simulink model "InAmpCode"  (R2025b)
settings: Solver=VariableStepAuto  StartTime=0.0  StopTime=10  RelTol=1e-3
libraries: fl_lib x15, nesl_utility x3
settings Model: Creator=Bassel  LastModifiedBy=Bassel

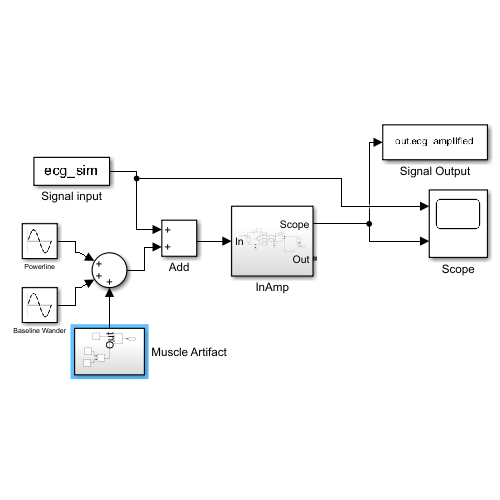
[thumbnail: Simulink's stored preview of the top-level diagram]
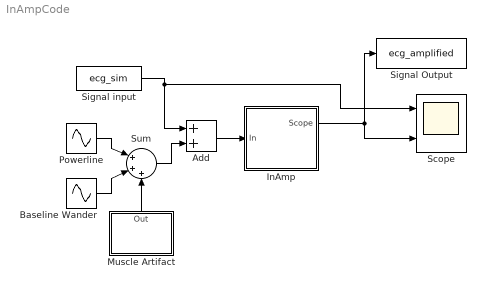
== system InAmpCode ==
  Add : Sum
  Baseline Wander : Sin  Amplitude=0.1  Frequency=0.2*2*pi  Phase=(pi/2)*2  SampleTime=0
  InAmp : Subsystem
  Muscle Artifact : Subsystem
  Powerline : Sin  Amplitude=0.1  Frequency=50*2*pi  SampleTime=0
  Scope : Scope  NumInputPorts=2
      settings: ActiveDisplayYMinimum=-0.24396112292352057  ActiveDisplayYMaximum=1.1258307290566818
  Signal Output : ToWorkspace  VariableName=ecg_amplified  SaveFormat=Timeseries  SampleTime=-1
  Signal input : FromWorkspace  VariableName=ecg_sim
  Sum : Sum  Inputs=|+++
  wires:
  Add/1 -> InAmp/1(In)
  Muscle Artifact/1(Out) -> Sum/3
  Signal input/1 -> Scope/1, Add/1
  Sum/1 -> Add/2
  Powerline/1 -> Sum/1
  Baseline Wander/1 -> Sum/2
  InAmp/1(Scope) -> Signal Output/1, Scope/2

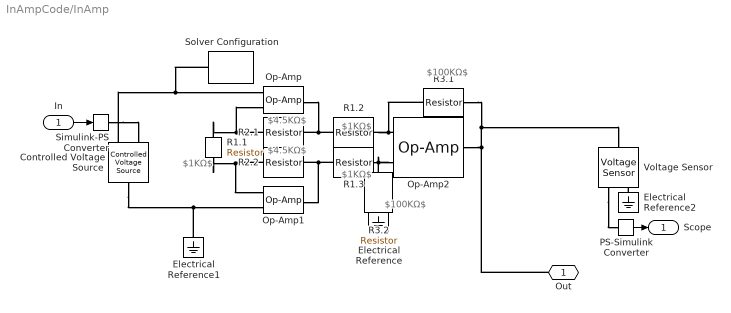
== system InAmpCode/InAmp ==
  note: $4.5KΩ$
  note: $1KΩ$
  note: $100KΩ$
  note: $100KΩ$
  note: $1KΩ$
  note: $1KΩ$
  note: $4.5KΩ$
  In : Inport
  Controlled Voltage Source : fl_lib/Electrical/Electrical Sources/Controlled Voltage Source
  Electrical Reference : fl_lib/Electrical/Electrical Elements/Electrical Reference
  Electrical Reference1 : fl_lib/Electrical/Electrical Elements/Electrical Reference
  Electrical Reference2 : fl_lib/Electrical/Electrical Elements/Electrical Reference
  Op-Amp : fl_lib/Electrical/Electrical Elements/Op-Amp  outI_specify=off  outI_priority=None  outI=0 A  outI_nominal_specify=off  outI_nominal_value=1  outI_nominal_unit=A
  Op-Amp1 : fl_lib/Electrical/Electrical Elements/Op-Amp  outI_specify=off  outI_priority=None  outI=0 A  outI_nominal_specify=off  outI_nominal_value=1  outI_nominal_unit=A
  Op-Amp2 : fl_lib/Electrical/Electrical Elements/Op-Amp  outI_specify=off  outI_priority=None  outI=0 A  outI_nominal_specify=off  outI_nominal_value=1  outI_nominal_unit=A
  PS-Simulink Converter : nesl_utility/PS-Simulink Converter  PhysicalDomain=network_engine_domain  SubClassName=ps_output  LeftPortType=input  RightPortType=output  PseudoPeriodic=off  Frequencies=[]  VectorFormat=inherit  Unit=inherit  AffineConversion=off
  R1.1 : fl_lib/Electrical/Electrical Elements/Resistor  R=1000 Ohm  i_specify=off  i_priority=None  i=0 A  i_nominal_specify=off  i_nominal_value=1  i_nominal_unit=A  v_specify=off  v_priority=None  v=0 V  v_nominal_specify=off  v_nominal_value=1  v_nominal_unit=V
  R1.2 : fl_lib/Electrical/Electrical Elements/Resistor  R=1000 Ohm  i_specify=off  i_priority=None  i=0 A  i_nominal_specify=off  i_nominal_value=1  i_nominal_unit=A  v_specify=off  v_priority=None  v=0 V  v_nominal_specify=off  v_nominal_value=1  v_nominal_unit=V
  R1.3 : fl_lib/Electrical/Electrical Elements/Resistor  R=1000 Ohm  i_specify=off  i_priority=None  i=0 A  i_nominal_specify=off  i_nominal_value=1  i_nominal_unit=A  v_specify=off  v_priority=None  v=0 V  v_nominal_specify=off  v_nominal_value=1  v_nominal_unit=V
  R2.1 : fl_lib/Electrical/Electrical Elements/Resistor  R=4500 Ohm  i_specify=off  i_priority=None  i=0 A  i_nominal_specify=off  i_nominal_value=1  i_nominal_unit=A  v_specify=off  v_priority=None  v=0 V  v_nominal_specify=off  v_nominal_value=1  v_nominal_unit=V
  R2.2 : fl_lib/Electrical/Electrical Elements/Resistor  R=4500 Ohm  i_specify=off  i_priority=None  i=0 A  i_nominal_specify=off  i_nominal_value=1  i_nominal_unit=A  v_specify=off  v_priority=None  v=0 V  v_nominal_specify=off  v_nominal_value=1  v_nominal_unit=V
  R3.1 : fl_lib/Electrical/Electrical Elements/Resistor  R=100000 Ohm  i_specify=off  i_priority=None  i=0 A  i_nominal_specify=off  i_nominal_value=1  i_nominal_unit=A  v_specify=off  v_priority=None  v=0 V  v_nominal_specify=off  v_nominal_value=1  v_nominal_unit=V
  R3.2 : fl_lib/Electrical/Electrical Elements/Resistor  R=100000 Ohm  i_specify=off  i_priority=None  i=0 A  i_nominal_specify=off  i_nominal_value=1  i_nominal_unit=A  v_specify=off  v_priority=None  v=0 V  v_nominal_specify=off  v_nominal_value=1  v_nominal_unit=V
  Simulink-PS Converter : nesl_utility/Simulink-PS Converter  PhysicalDomain=network_engine_domain  SubClassName=ps_input  LeftPortType=input  RightPortType=output  PseudoPeriodic=off  Frequencies=[]  NoiseDistribution=none  NoiseParameters=[]  Unit=1  AffineConversion=off  FilteringAndDerivatives=provide  SimscapeFilterOrder=1  InputFilterTimeConstant=0.001  UdotUserProvided=0
  Solver Configuration : nesl_utility/Solver Configuration  PhysicalDomain=network_engine_domain  SubClassName=solver  LeftPortType=input  RightPortType=generic  Tones=[]  Harmonics=[]  SimulateNoise=off  Profile=off  UseLocalSampling=off  EnableSwitchedLinearOptims=on  FrequencyDomain=off  UseCCode=off  RelTol=0.001  AbsTol=0.001  MinStep=1e-09  ToWorkspace=off  RevertToSquareIcSolve=off  NumHomotopyIterations=100  PhasorMode=off  PhasorModeNumHarmonics=1  ConsistencySolver=NEWTON_XTOL_AFTER_FTOL  IndexReductionMethod=DerivativeReplacement  DoDC=off  ResidualTolerance=1e-09  ConsistencyTolSource=GLOBAL  ConsistencyAbsTol=0.001  ConsistencyRelTol=0.001  ConsistencyTolFactor=0.001  UseLocalSolver=off  LocalSolverChoice=NE_BACKWARD_EULER_ADVANCER  ResolveIndetEquations=on  FunctionEvalNumThread=1  LocalSolverSampleTime=0.001  DoFixedCost=off  MaxNonlinIter=3  MaxModeIter=2  ComputeImpulses=off  ImpulseIterations=2  LinearAlgebra=auto  LinearAlgebraNumThread=0  EquationFormulation=NE_TIME_EF  DelaysMemoryBudget=1024  AutomaticFiltering=on  FilteringTimeConstant=0.001  PartitionStorageMethod=AS_NEEDED  PartitionMemoryBudget=1024  PartitionMethod=ROBUST  MultibodyUseLocalSolver=off  MultibodyLocalSolverChoice=ODE1  MultibodyLocalSolverSampleTime=0.001
  Voltage Sensor : fl_lib/Electrical/Electrical Sensors/Voltage Sensor
  Out : PMIOPort  Side=Right
  Scope : Outport
  wires:
  In/1 -> Simulink-PS Converter/1
  PS-Simulink Converter/1 -> Scope/1
  connections:
  R2.1/LConn1 -- R1.1/LConn1 -- Op-Amp/LConn2
  Op-Amp1/RConn1 -- R1.3/LConn1 -- R2.2/RConn1
  Op-Amp2/LConn2 -- R3.1/LConn1 -- R1.2/RConn1
  Op-Amp2/RConn1 -- R3.1/RConn1 -- Voltage Sensor/LConn1 -- Out/RConn1
  R2.2/LConn1 -- R1.1/RConn1 -- Op-Amp1/LConn2
  R1.3/RConn1 -- R3.2/LConn1 -- Op-Amp2/LConn1
  Electrical Reference1/LConn1 -- Op-Amp1/LConn1 -- Controlled Voltage Source/LConn1
  Electrical Reference/LConn1 -- R3.2/RConn1
  Solver Configuration/RConn1 -- Op-Amp/LConn1 -- Controlled Voltage Source/RConn2
  Op-Amp/RConn1 -- R1.2/LConn1 -- R2.1/RConn1
  Voltage Sensor/RConn1 -- PS-Simulink Converter/LConn1
  Electrical Reference2/LConn1 -- Voltage Sensor/RConn2
  Simulink-PS Converter/RConn1 -- Controlled Voltage Source/RConn1

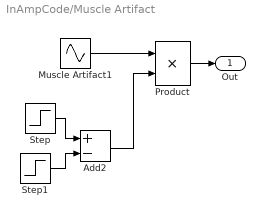
== system InAmpCode/Muscle Artifact ==
  Add2 : Sum  Inputs=+-
  Muscle Artifact1 : Sin  Amplitude=0.3  Frequency=45*2*pi  SampleTime=0  VectorParams1D=off
  Product : Product
  Step : Step  Time=5.25  SampleTime=0
  Step1 : Step  Time=6.25  SampleTime=0
  Out : Outport
  wires:
  Product/1 -> Out/1
  Step/1 -> Add2/1
  Step1/1 -> Add2/2
  Add2/1 -> Product/2
  Muscle Artifact1/1 -> Product/1
